simulink model "dig_int_kurt"  (Simulink 6.2)
settings: Solver=ode45  StartTime=0.0  StopTime=1  RelTol=1e-3
undefined symbols (not defined in the file): bit_rev, iBOB, pfb_coeff_gen_calc
libraries: xbsIndex_r3 x1084, casper_library x95, xps_library x32
(part 6 of 8)

== system dig_int_kurt/fft/fft_biplex0/biplex_core/fft_stage_9 ==
  in1 : Inport  Port=1  LatchInput=off
  in2 : Inport  Port=2  LatchInput=off
  of_in : Inport  Port=3  LatchInput=off
  sync : Inport  Port=4  LatchInput=off
  shift : Inport  Port=5  LatchInput=off
  Counter : xbsIndex_r3/Counter  cnt_type=Free Running  n_bits=FFTSize-FFTStage+1  bin_pt=0  arith_type=Unsigned  start_count=0  cnt_to=Inf  cnt_by_val=1  operation=Up  explicit_period=off  period=1  load_pin=off  rst=on  en=off  dbl_ovrd=off  show_param=off  use_rpm=off  gen_core=on
      settings: xl_area=[0, 0, 0, 0, 0, 0, 0]
  Delay : xbsIndex_r3/Delay  latency=1  reg_retiming=off  explicit_period=off  period=1  en=off  accept_only_valid=off  init_zero=on  dbl_ovrd=off  show_param=off
      settings: xl_area=[0, 0, 0, 0, 0, 0, 0]
  Logical1 : xbsIndex_r3/Logical  logical_function=OR  inputs=2  precision=Full  arith_type=Unsigned  n_bits=8  bin_pt=2  align_bp=on  latency=1  explicit_period=on  period=1  en=off  dbl_ovrd=off  show_param=off
      settings: xl_area=[0, 0, 0, 0, 0, 0, 0]
  Mux : xbsIndex_r3/Mux  inputs=2  precision=Full  arith_type="Signed  (2's comp)"  n_bits=8  bin_pt=2  quantization=Truncate  overflow=Wrap  latency=1  explicit_period=off  period=1  en=off  dbl_ovrd=off  show_param=off  mux_type=off  use_rpm=off  gen_core=on
      settings: xl_area=[0, 0, 0, 0, 0, 0, 0]
  Mux1 : xbsIndex_r3/Mux  inputs=2  precision=Full  arith_type="Signed  (2's comp)"  n_bits=8  bin_pt=2  quantization=Truncate  overflow=Wrap  latency=1  explicit_period=off  period=1  en=off  dbl_ovrd=off  show_param=off  mux_type=off  use_rpm=off  gen_core=on
      settings: xl_area=[0, 0, 0, 0, 0, 0, 0]
  Slice : xbsIndex_r3/Slice  Orientation=up  mode=Lower Bit Location + Width  nbits=1  bit1=-(FFTStage - 1)  base1=MSB of Input  bit0=FFTStage - 1  base0=LSB of Input  boolean_output=on  explicit_period=off  period=1  dbl_ovrd=off
  Slice1 : xbsIndex_r3/Slice  mode=Upper Bit Location + Width  nbits=1  bit1=0  base1=MSB of Input  bit0=0  base0=LSB of Input  boolean_output=off  explicit_period=off  period=1  dbl_ovrd=off
  butterfly_direct : Subsystem  AncestorBlock=casper_library/FFTs/butterfly_direct  mask(butterfly_direct){FFTSize=10, Coeffs=getfield( getfield( get_param( gcb,'UserData'), 'parameters'),'Coeffs'), StepPeriod=1, BitWidth=18, add_latency=3, mult_latency=4, bram_latency=3, use_bram=0, quantization=Truncate, overflow=Wrap}
      mask prompts: FFTSize "Size of FFT: (2^?)"; Coeffs "Coefficients: (0 to 2^(FFTSize-1)-1)"; StepPeriod "Coefficient Step Period: (2^?)"; BitWidth "Output Bitwidth:"; add_latency "Add Latency"; mult_latency "Mult Latency"; bram_latency "BRAM Latency"; use_bram "Store Coefficients in BRAM"; quantization "Quantization Behavior"; overflow "Overflow Behavior"
      mask init: same as dig_int_kurt/fft/fft_biplex0/biplex_core/fft_stage_10/butterfly_direct
      settings: AttributesFormatString=|
      | FFTSize=10, Coeffs=[0    1    2    3    4    5    6    7    8    9   10   11   12   13   14   15   16   17   18   19   20   21   22   23   24   25   26   27   28   29   30   31   32   33   34   35   36   37   38   39   40   41   42   43   44   45   46   47   48   49   50   51   52   53   54   55   56   57   58   59   60   61   62   63   64   65   66   67   68   69   70   71   72   73   74   75   76   77   78   79   80   81   82   83   84   85   86   87   88   89   90   91   92   93   94   95   96   97   98   99  100  101  102  103  104  105  106  107  108  109  110  111  112  113  114  115  116  117  118  119  120  121  122  123  124  125  126  127  128  129  130  131  132  133  134  135  136  137  138  139  140  141  142  143  144  145  146  147  148  149  150  151  152  153  154  155  156  157  158  159  160  161  162  163  164  165  166  167  168  169  170  171  172  173  174  175  176  177  178  179  180  181  182  183  184  185  186  187  188  189  190  191  192  193  194  195  196  197  198  199  200  201  202  203  204  205  206  207  208  209  210  211  212  213  214  215  216  217  218  219  220  221  222  223  224  225  226  227  228  229  230  231  232  233  234  235  236  237  238  239  240  241  242  243  244  245  246  247  248  249  250  251  252  253  254  255],
      |  StepPeriod=1, BitWidth=18
      mask StyleString: edit,edit,edit,edit,edit,edit,edit,edit,popup(Truncate|Round  (unbiased: +/- Inf)|Round  (unbiased: Even Values)),popup(Wrap|Saturate|Error)
  delay_b : Subsystem  BlockChoice=delay_slr
      link override delay_bram: bram_latency=bram_latency  DelayLen=2^(FFTSize-FFTStage)
      link override delay_slr: DelayLen=2^(FFTSize-FFTStage)
      settings: AttributesFormatString=%<BlockChoice>  TemplateBlock=casper_library/Delays/delay  MemberBlocks=delay_bram,delay_slr
  delay_f : Subsystem  BlockChoice=delay_slr
      link override delay_bram: bram_latency=bram_latency  DelayLen=2^(FFTSize-FFTStage)
      link override delay_slr: DelayLen=2^(FFTSize-FFTStage)
      settings: AttributesFormatString=%<BlockChoice>  TemplateBlock=casper_library/Delays/delay  MemberBlocks=delay_bram,delay_slr
  sync_delay : casper_library/Delays/sync_delay  DelayLen=2^(FFTSize - FFTStage)
      link override Constant: equ=P=C
      link override Constant1: equ=P=C
      link override Constant2: equ=P=C
      link override Constant3: equ=P=C
  out1 : Outport
  out2 : Outport  Port=2
  of : Outport  Port=3
  sync_out : Outport  Port=4
  wires:
  butterfly_direct/4(sync_out) -> sync_out/1
  butterfly_direct/1(a+bw) -> out1/1
  butterfly_direct/2(a-bw) -> out2/1
  butterfly_direct/3(of) -> Logical1/1
  Slice/1 -> butterfly_direct/4(shift)
  sync_delay/1 -> butterfly_direct/3(sync)
  delay_b/1(Out1) -> butterfly_direct/1(a)
  in2/1 -> delay_f/1(In1)
  Slice1/1 -> Mux1/1, Mux/1
  in1/1 -> Mux1/2, Mux/3
  delay_f/1(Out1) -> Mux/2, Mux1/3
  Mux1/1 -> delay_b/1(In1)
  Mux/1 -> butterfly_direct/2(b)
  Counter/1 -> Slice1/1
  sync/1 -> Delay/1, Counter/1
  Delay/1 -> sync_delay/1
  Logical1/1 -> of/1
  of_in/1 -> Logical1/2
  shift/1 -> Slice/1

== system dig_int_kurt/fft/fft_biplex0/biplex_cplx_unscrambler/barrel_switcher ==
  sel : Inport  Port=1  LatchInput=off
  sync_in : Inport  Port=2  LatchInput=off
  In1 : Inport  Port=3  LatchInput=off
  In2 : Inport  Port=4  LatchInput=off
  Delay_sync : xbsIndex_r3/Delay  latency=1  reg_retiming=off  explicit_period=off  period=1  en=off  accept_only_valid=off  init_zero=on  dbl_ovrd=off  show_param=off
      settings: xl_area=[0, 0, 0, 0, 0, 0, 0]
  Mux11 : xbsIndex_r3/Mux  inputs=2  precision=Full  arith_type="Signed  (2's comp)"  n_bits=8  bin_pt=2  quantization=Truncate  overflow=Wrap  latency=1  explicit_period=off  period=1  en=off  dbl_ovrd=off  show_param=off  mux_type=off  use_rpm=off  gen_core=off
      settings: xl_area=[0, 0, 0, 0, 0, 0, 0]
  Mux21 : xbsIndex_r3/Mux  inputs=2  precision=Full  arith_type="Signed  (2's comp)"  n_bits=8  bin_pt=2  quantization=Truncate  overflow=Wrap  latency=1  explicit_period=off  period=1  en=off  dbl_ovrd=off  show_param=off  mux_type=off  use_rpm=off  gen_core=off
      settings: xl_area=[0, 0, 0, 0, 0, 0, 0]
  Slice1 : xbsIndex_r3/Slice  mode=Upper Bit Location + Width  nbits=1  bit1=-0  base1=MSB of Input  bit0=0  base0=LSB of Input  boolean_output=off  explicit_period=off  period=1  dbl_ovrd=off
  sync_out : Outport
  Out1 : Outport  Port=2
  Out2 : Outport  Port=3
  wires:
  sync_in/1 -> Delay_sync/1
  Delay_sync/1 -> sync_out/1
  sel/1 -> Slice1/1
  Slice1/1 -> Mux11/1, Mux21/1
  In1/1 -> Mux11/2, Mux21/3
  Mux11/1 -> Out1/1
  In2/1 -> Mux21/2, Mux11/3
  Mux21/1 -> Out2/1

== system dig_int_kurt/fft/fft_biplex0/biplex_cplx_unscrambler/barrel_switcher1 ==
  sel : Inport  Port=1  LatchInput=off
  sync_in : Inport  Port=2  LatchInput=off
  In1 : Inport  Port=3  LatchInput=off
  In2 : Inport  Port=4  LatchInput=off
  Delay_sync : xbsIndex_r3/Delay  latency=1  reg_retiming=off  explicit_period=off  period=1  en=off  accept_only_valid=off  init_zero=on  dbl_ovrd=off  show_param=off
      settings: xl_area=[0, 0, 0, 0, 0, 0, 0]
  Mux11 : xbsIndex_r3/Mux  inputs=2  precision=Full  arith_type="Signed  (2's comp)"  n_bits=8  bin_pt=2  quantization=Truncate  overflow=Wrap  latency=1  explicit_period=off  period=1  en=off  dbl_ovrd=off  show_param=off  mux_type=off  use_rpm=off  gen_core=off
      settings: xl_area=[0, 0, 0, 0, 0, 0, 0]
  Mux21 : xbsIndex_r3/Mux  inputs=2  precision=Full  arith_type="Signed  (2's comp)"  n_bits=8  bin_pt=2  quantization=Truncate  overflow=Wrap  latency=1  explicit_period=off  period=1  en=off  dbl_ovrd=off  show_param=off  mux_type=off  use_rpm=off  gen_core=off
      settings: xl_area=[0, 0, 0, 0, 0, 0, 0]
  Slice1 : xbsIndex_r3/Slice  mode=Upper Bit Location + Width  nbits=1  bit1=-0  base1=MSB of Input  bit0=0  base0=LSB of Input  boolean_output=off  explicit_period=off  period=1  dbl_ovrd=off
  sync_out : Outport
  Out1 : Outport  Port=2
  Out2 : Outport  Port=3
  wires:
  sync_in/1 -> Delay_sync/1
  Delay_sync/1 -> sync_out/1
  sel/1 -> Slice1/1
  Slice1/1 -> Mux11/1, Mux21/1
  In1/1 -> Mux11/2, Mux21/3
  Mux11/1 -> Out1/1
  In2/1 -> Mux21/2, Mux11/3
  Mux21/1 -> Out2/1

== system dig_int_kurt/fft/fft_biplex0/biplex_cplx_unscrambler/reorder ==
  sync : Inport  Port=1  LatchInput=off
  en : Inport  Port=2  LatchInput=off
  din0 : Inport  Port=3  LatchInput=off
  Counter : xbsIndex_r3/Counter  cnt_type=Count Limited  n_bits=11  bin_pt=0  arith_type=Unsigned  start_count=0  cnt_to=2047  cnt_by_val=1  operation=Up  explicit_period=off  period=1  load_pin=off  rst=on  en=on  dbl_ovrd=off  show_param=off  use_rpm=on  gen_core=off
      settings: xl_area=[0, 0, 0, 0, 0, 0, 0]
  Mux : xbsIndex_r3/Mux  inputs=2  precision=Full  arith_type="Signed  (2's comp)"  n_bits=8  bin_pt=2  quantization=Truncate  overflow=Wrap  latency=1  explicit_period=off  period=1  en=off  dbl_ovrd=off  show_param=off  mux_type=off  use_rpm=off  gen_core=off
      settings: xl_area=[0, 0, 0, 0, 0, 0, 0]
  Slice1 : xbsIndex_r3/Slice  mode=Upper Bit Location + Width  nbits=1  bit1=0  base1=MSB of Input  bit0=0  base0=LSB of Input  boolean_output=off  explicit_period=off  period=1  dbl_ovrd=off
  Slice2 : xbsIndex_r3/Slice  mode=Lower Bit Location + Width  nbits=10  bit1=0  base1=MSB of Input  bit0=0  base0=LSB of Input  boolean_output=off  explicit_period=off  period=1  dbl_ovrd=off
  bram0 : xbsIndex_r3/Single Port RAM  depth=1024  initVector=sin(pi*(0:15)/16)  write_mode=Read Before Write  latency=3  init_zero=on  explicit_period=off  period=1  rst=off  init_reg=0  en=off  dbl_ovrd=off  show_param=off  distributed_mem=off  use_rpm=off  gen_core=off
      settings: xl_area=[0, 0, 0, 0, 0, 0, 0]
  delay_d0 : xbsIndex_r3/Delay  latency=0  reg_retiming=off  explicit_period=off  period=1  en=off  accept_only_valid=off  init_zero=on  dbl_ovrd=off  show_param=off
      settings: xl_area=[0, 0, 0, 0, 0, 0, 0]
  delay_din0 : xbsIndex_r3/Delay  latency=1  reg_retiming=off  explicit_period=off  period=1  en=off  accept_only_valid=off  init_zero=on  dbl_ovrd=off  show_param=off
      settings: xl_area=[0, 0, 0, 0, 0, 0, 0]
  delay_map1 : xbsIndex_r3/Delay  latency=0*map_latency  reg_retiming=off  explicit_period=off  period=1  en=off  accept_only_valid=off  init_zero=on  dbl_ovrd=off  show_param=off
      settings: xl_area=[0, 0, 0, 0, 0, 0, 0]
  delay_sel : xbsIndex_r3/Delay  latency=0  reg_retiming=off  explicit_period=off  period=1  en=off  accept_only_valid=off  init_zero=on  dbl_ovrd=off  show_param=off
      settings: xl_area=[0, 0, 0, 0, 0, 0, 0]
  delay_valid : xbsIndex_r3/Delay  latency=4  reg_retiming=off  explicit_period=off  period=1  en=off  accept_only_valid=off  init_zero=on  dbl_ovrd=off  show_param=off
      settings: xl_area=[0, 0, 0, 0, 0, 0, 0]
  delay_we : xbsIndex_r3/Delay  latency=0  reg_retiming=off  explicit_period=off  period=1  en=off  accept_only_valid=off  init_zero=on  dbl_ovrd=off  show_param=off
      settings: xl_area=[0, 0, 0, 0, 0, 0, 0]
  map1 : Subsystem  AncestorBlock=casper_library/FFTs/map  mask(map){map=getfield( getfield( get_param( gcb,'UserData'), 'parameters'),'map'), latency=0}
      mask init:
      | map_init(gcb, 'map', map, 'latency', latency)
  post_sync_delay : xbsIndex_r3/Delay  latency=4  reg_retiming=off  explicit_period=off  period=1  en=off  accept_only_valid=off  init_zero=on  dbl_ovrd=off  show_param=off
      settings: xl_area=[0, 0, 0, 0, 0, 0, 0]
  pre_sync_delay : xbsIndex_r3/Delay  latency=0  reg_retiming=off  explicit_period=off  period=1  en=off  accept_only_valid=off  init_zero=on  dbl_ovrd=off  show_param=off
      settings: xl_area=[0, 0, 0, 0, 0, 0, 0]
  sync_delay_en : casper_library/Delays/sync_delay_en  DelayLen=1024
      link override Constant: equ=P=C
      link override Constant1: equ=P=C
      link override Constant2: equ=P=C
      link override Constant3: equ=P=C
  sync_out : Outport
  valid : Outport  Port=2
  dout0 : Outport  Port=3
  wires:
  sync/1 -> Counter/1, pre_sync_delay/1
  en/1 -> Counter/2, sync_delay_en/2, delay_we/1
  Counter/1 -> Slice1/1, Slice2/1
  Slice1/1 -> delay_sel/1
  delay_sel/1 -> Mux/1
  Slice2/1 -> delay_d0/1, map1/1(din)
  delay_d0/1 -> Mux/2
  pre_sync_delay/1 -> sync_delay_en/1
  sync_delay_en/1 -> post_sync_delay/1
  post_sync_delay/1 -> sync_out/1
  delay_we/1 -> delay_valid/1, bram0/3
  delay_valid/1 -> valid/1
  Mux/1 -> bram0/1
  din0/1 -> delay_din0/1
  delay_din0/1 -> bram0/2
  bram0/1 -> dout0/1
  map1/1(dout) -> delay_map1/1
  delay_map1/1 -> Mux/3

== system dig_int_kurt/fft/fft_biplex0/biplex_cplx_unscrambler/reorder1 ==
  sync : Inport  Port=1  LatchInput=off
  en : Inport  Port=2  LatchInput=off
  din0 : Inport  Port=3  LatchInput=off
  Counter : xbsIndex_r3/Counter  cnt_type=Count Limited  n_bits=11  bin_pt=0  arith_type=Unsigned  start_count=0  cnt_to=2047  cnt_by_val=1  operation=Up  explicit_period=off  period=1  load_pin=off  rst=on  en=on  dbl_ovrd=off  show_param=off  use_rpm=on  gen_core=off
      settings: xl_area=[0, 0, 0, 0, 0, 0, 0]
  Mux : xbsIndex_r3/Mux  inputs=2  precision=Full  arith_type="Signed  (2's comp)"  n_bits=8  bin_pt=2  quantization=Truncate  overflow=Wrap  latency=1  explicit_period=off  period=1  en=off  dbl_ovrd=off  show_param=off  mux_type=off  use_rpm=off  gen_core=off
      settings: xl_area=[0, 0, 0, 0, 0, 0, 0]
  Slice1 : xbsIndex_r3/Slice  mode=Upper Bit Location + Width  nbits=1  bit1=0  base1=MSB of Input  bit0=0  base0=LSB of Input  boolean_output=off  explicit_period=off  period=1  dbl_ovrd=off
  Slice2 : xbsIndex_r3/Slice  mode=Lower Bit Location + Width  nbits=10  bit1=0  base1=MSB of Input  bit0=0  base0=LSB of Input  boolean_output=off  explicit_period=off  period=1  dbl_ovrd=off
  bram0 : xbsIndex_r3/Single Port RAM  depth=1024  initVector=sin(pi*(0:15)/16)  write_mode=Read Before Write  latency=3  init_zero=on  explicit_period=off  period=1  rst=off  init_reg=0  en=off  dbl_ovrd=off  show_param=off  distributed_mem=off  use_rpm=off  gen_core=off
      settings: xl_area=[0, 0, 0, 0, 0, 0, 0]
  delay_d0 : xbsIndex_r3/Delay  latency=0  reg_retiming=off  explicit_period=off  period=1  en=off  accept_only_valid=off  init_zero=on  dbl_ovrd=off  show_param=off
      settings: xl_area=[0, 0, 0, 0, 0, 0, 0]
  delay_din0 : xbsIndex_r3/Delay  latency=1  reg_retiming=off  explicit_period=off  period=1  en=off  accept_only_valid=off  init_zero=on  dbl_ovrd=off  show_param=off
      settings: xl_area=[0, 0, 0, 0, 0, 0, 0]
  delay_map1 : xbsIndex_r3/Delay  latency=0*map_latency  reg_retiming=off  explicit_period=off  period=1  en=off  accept_only_valid=off  init_zero=on  dbl_ovrd=off  show_param=off
      settings: xl_area=[0, 0, 0, 0, 0, 0, 0]
  delay_sel : xbsIndex_r3/Delay  latency=0  reg_retiming=off  explicit_period=off  period=1  en=off  accept_only_valid=off  init_zero=on  dbl_ovrd=off  show_param=off
      settings: xl_area=[0, 0, 0, 0, 0, 0, 0]
  delay_valid : xbsIndex_r3/Delay  latency=4  reg_retiming=off  explicit_period=off  period=1  en=off  accept_only_valid=off  init_zero=on  dbl_ovrd=off  show_param=off
      settings: xl_area=[0, 0, 0, 0, 0, 0, 0]
  delay_we : xbsIndex_r3/Delay  latency=0  reg_retiming=off  explicit_period=off  period=1  en=off  accept_only_valid=off  init_zero=on  dbl_ovrd=off  show_param=off
      settings: xl_area=[0, 0, 0, 0, 0, 0, 0]
  map1 : Subsystem  AncestorBlock=casper_library/FFTs/map  mask(map){map=getfield( getfield( get_param( gcb,'UserData'), 'parameters'),'map'), latency=0}
      mask init:
      | map_init(gcb, 'map', map, 'latency', latency)
  post_sync_delay : xbsIndex_r3/Delay  latency=4  reg_retiming=off  explicit_period=off  period=1  en=off  accept_only_valid=off  init_zero=on  dbl_ovrd=off  show_param=off
      settings: xl_area=[0, 0, 0, 0, 0, 0, 0]
  pre_sync_delay : xbsIndex_r3/Delay  latency=0  reg_retiming=off  explicit_period=off  period=1  en=off  accept_only_valid=off  init_zero=on  dbl_ovrd=off  show_param=off
      settings: xl_area=[0, 0, 0, 0, 0, 0, 0]
  sync_delay_en : casper_library/Delays/sync_delay_en  DelayLen=1024
      link override Constant: equ=P=C
      link override Constant1: equ=P=C
      link override Constant2: equ=P=C
      link override Constant3: equ=P=C
  sync_out : Outport
  valid : Outport  Port=2
  dout0 : Outport  Port=3
  wires:
  sync/1 -> Counter/1, pre_sync_delay/1
  en/1 -> Counter/2, sync_delay_en/2, delay_we/1
  Counter/1 -> Slice1/1, Slice2/1
  Slice1/1 -> delay_sel/1
  delay_sel/1 -> Mux/1
  Slice2/1 -> delay_d0/1, map1/1(din)
  delay_d0/1 -> Mux/2
  pre_sync_delay/1 -> sync_delay_en/1
  sync_delay_en/1 -> post_sync_delay/1
  post_sync_delay/1 -> sync_out/1
  delay_we/1 -> delay_valid/1, bram0/3
  delay_valid/1 -> valid/1
  Mux/1 -> bram0/1
  din0/1 -> delay_din0/1
  delay_din0/1 -> bram0/2
  bram0/1 -> dout0/1
  map1/1(dout) -> delay_map1/1
  delay_map1/1 -> Mux/3

== system dig_int_kurt/pfb_fir/pol1_in1_last_tap/pfb_add_tree/adder_tree1 ==
  sync : Inport  Port=1  LatchInput=off
  din1 : Inport  Port=2  LatchInput=off
  din2 : Inport  Port=3  LatchInput=off
  din3 : Inport  Port=4  LatchInput=off
  din4 : Inport  Port=5  LatchInput=off
  addr1 : xbsIndex_r3/AddSub  mode=Addition  precision=Full  arith_type=Unsigned  n_bits=8  bin_pt=2  quantization=Truncate  overflow=Wrap  latency=2  explicit_period=off  period=1  use_carryin=off  use_carryout=off  en=off  dbl_ovrd=off  show_param=off  use_core=on  pipeline=on  use_rpm=on  gen_core=off
      settings: xl_area=[0, 0, 0, 0, 0, 0, 0]
  addr2 : xbsIndex_r3/AddSub  mode=Addition  precision=Full  arith_type=Unsigned  n_bits=8  bin_pt=2  quantization=Truncate  overflow=Wrap  latency=2  explicit_period=off  period=1  use_carryin=off  use_carryout=off  en=off  dbl_ovrd=off  show_param=off  use_core=on  pipeline=on  use_rpm=on  gen_core=off
      settings: xl_area=[0, 0, 0, 0, 0, 0, 0]
  addr3 : xbsIndex_r3/AddSub  mode=Addition  precision=Full  arith_type=Unsigned  n_bits=8  bin_pt=2  quantization=Truncate  overflow=Wrap  latency=2  explicit_period=off  period=1  use_carryin=off  use_carryout=off  en=off  dbl_ovrd=off  show_param=off  use_core=on  pipeline=on  use_rpm=on  gen_core=off
      settings: xl_area=[0, 0, 0, 0, 0, 0, 0]
  sync_delay : xbsIndex_r3/Delay  latency=4  reg_retiming=off  explicit_period=off  period=1  en=off  accept_only_valid=off  init_zero=on  dbl_ovrd=off  show_param=off
      settings: xl_area=[0, 0, 0, 0, 0, 0, 0]
  sync_out : Outport
  dout : Outport  Port=2
  wires:
  sync/1 -> sync_delay/1
  sync_delay/1 -> sync_out/1
  din1/1 -> addr1/1
  din2/1 -> addr1/2
  din3/1 -> addr2/1
  din4/1 -> addr2/2
  addr1/1 -> addr3/1
  addr2/1 -> addr3/2
  addr3/1 -> dout/1

== system dig_int_kurt/pfb_fir/pol1_in1_last_tap/pfb_add_tree/adder_tree2 ==
  sync : Inport  Port=1  LatchInput=off
  din1 : Inport  Port=2  LatchInput=off
  din2 : Inport  Port=3  LatchInput=off
  din3 : Inport  Port=4  LatchInput=off
  din4 : Inport  Port=5  LatchInput=off
  addr1 : xbsIndex_r3/AddSub  mode=Addition  precision=Full  arith_type=Unsigned  n_bits=8  bin_pt=2  quantization=Truncate  overflow=Wrap  latency=2  explicit_period=off  period=1  use_carryin=off  use_carryout=off  en=off  dbl_ovrd=off  show_param=off  use_core=on  pipeline=on  use_rpm=on  gen_core=off
      settings: xl_area=[0, 0, 0, 0, 0, 0, 0]
  addr2 : xbsIndex_r3/AddSub  mode=Addition  precision=Full  arith_type=Unsigned  n_bits=8  bin_pt=2  quantization=Truncate  overflow=Wrap  latency=2  explicit_period=off  period=1  use_carryin=off  use_carryout=off  en=off  dbl_ovrd=off  show_param=off  use_core=on  pipeline=on  use_rpm=on  gen_core=off
      settings: xl_area=[0, 0, 0, 0, 0, 0, 0]
  addr3 : xbsIndex_r3/AddSub  mode=Addition  precision=Full  arith_type=Unsigned  n_bits=8  bin_pt=2  quantization=Truncate  overflow=Wrap  latency=2  explicit_period=off  period=1  use_carryin=off  use_carryout=off  en=off  dbl_ovrd=off  show_param=off  use_core=on  pipeline=on  use_rpm=on  gen_core=off
      settings: xl_area=[0, 0, 0, 0, 0, 0, 0]
  sync_delay : xbsIndex_r3/Delay  latency=4  reg_retiming=off  explicit_period=off  period=1  en=off  accept_only_valid=off  init_zero=on  dbl_ovrd=off  show_param=off
      settings: xl_area=[0, 0, 0, 0, 0, 0, 0]
  sync_out : Outport
  dout : Outport  Port=2
  wires:
  sync/1 -> sync_delay/1
  sync_delay/1 -> sync_out/1
  din1/1 -> addr1/1
  din2/1 -> addr1/2
  din3/1 -> addr2/1
  din4/1 -> addr2/2
  addr1/1 -> addr3/1
  addr2/1 -> addr3/2
  addr3/1 -> dout/1

== system dig_int_kurt/pfb_fir/pol2_in1_last_tap/pfb_add_tree/adder_tree1 ==
  sync : Inport  Port=1  LatchInput=off
  din1 : Inport  Port=2  LatchInput=off
  din2 : Inport  Port=3  LatchInput=off
  din3 : Inport  Port=4  LatchInput=off
  din4 : Inport  Port=5  LatchInput=off
  addr1 : xbsIndex_r3/AddSub  mode=Addition  precision=Full  arith_type=Unsigned  n_bits=8  bin_pt=2  quantization=Truncate  overflow=Wrap  latency=2  explicit_period=off  period=1  use_carryin=off  use_carryout=off  en=off  dbl_ovrd=off  show_param=off  use_core=on  pipeline=on  use_rpm=on  gen_core=off
      settings: xl_area=[0, 0, 0, 0, 0, 0, 0]
  addr2 : xbsIndex_r3/AddSub  mode=Addition  precision=Full  arith_type=Unsigned  n_bits=8  bin_pt=2  quantization=Truncate  overflow=Wrap  latency=2  explicit_period=off  period=1  use_carryin=off  use_carryout=off  en=off  dbl_ovrd=off  show_param=off  use_core=on  pipeline=on  use_rpm=on  gen_core=off
      settings: xl_area=[0, 0, 0, 0, 0, 0, 0]
  addr3 : xbsIndex_r3/AddSub  mode=Addition  precision=Full  arith_type=Unsigned  n_bits=8  bin_pt=2  quantization=Truncate  overflow=Wrap  latency=2  explicit_period=off  period=1  use_carryin=off  use_carryout=off  en=off  dbl_ovrd=off  show_param=off  use_core=on  pipeline=on  use_rpm=on  gen_core=off
      settings: xl_area=[0, 0, 0, 0, 0, 0, 0]
  sync_delay : xbsIndex_r3/Delay  latency=4  reg_retiming=off  explicit_period=off  period=1  en=off  accept_only_valid=off  init_zero=on  dbl_ovrd=off  show_param=off
      settings: xl_area=[0, 0, 0, 0, 0, 0, 0]
  sync_out : Outport
  dout : Outport  Port=2
  wires:
  sync/1 -> sync_delay/1
  sync_delay/1 -> sync_out/1
  din1/1 -> addr1/1
  din2/1 -> addr1/2
  din3/1 -> addr2/1
  din4/1 -> addr2/2
  addr1/1 -> addr3/1
  addr2/1 -> addr3/2
  addr3/1 -> dout/1

== system dig_int_kurt/pfb_fir/pol2_in1_last_tap/pfb_add_tree/adder_tree2 ==
  sync : Inport  Port=1  LatchInput=off
  din1 : Inport  Port=2  LatchInput=off
  din2 : Inport  Port=3  LatchInput=off
  din3 : Inport  Port=4  LatchInput=off
  din4 : Inport  Port=5  LatchInput=off
  addr1 : xbsIndex_r3/AddSub  mode=Addition  precision=Full  arith_type=Unsigned  n_bits=8  bin_pt=2  quantization=Truncate  overflow=Wrap  latency=2  explicit_period=off  period=1  use_carryin=off  use_carryout=off  en=off  dbl_ovrd=off  show_param=off  use_core=on  pipeline=on  use_rpm=on  gen_core=off
      settings: xl_area=[0, 0, 0, 0, 0, 0, 0]
  addr2 : xbsIndex_r3/AddSub  mode=Addition  precision=Full  arith_type=Unsigned  n_bits=8  bin_pt=2  quantization=Truncate  overflow=Wrap  latency=2  explicit_period=off  period=1  use_carryin=off  use_carryout=off  en=off  dbl_ovrd=off  show_param=off  use_core=on  pipeline=on  use_rpm=on  gen_core=off
      settings: xl_area=[0, 0, 0, 0, 0, 0, 0]
  addr3 : xbsIndex_r3/AddSub  mode=Addition  precision=Full  arith_type=Unsigned  n_bits=8  bin_pt=2  quantization=Truncate  overflow=Wrap  latency=2  explicit_period=off  period=1  use_carryin=off  use_carryout=off  en=off  dbl_ovrd=off  show_param=off  use_core=on  pipeline=on  use_rpm=on  gen_core=off
      settings: xl_area=[0, 0, 0, 0, 0, 0, 0]
  sync_delay : xbsIndex_r3/Delay  latency=4  reg_retiming=off  explicit_period=off  period=1  en=off  accept_only_valid=off  init_zero=on  dbl_ovrd=off  show_param=off
      settings: xl_area=[0, 0, 0, 0, 0, 0, 0]
  sync_out : Outport
  dout : Outport  Port=2
  wires:
  sync/1 -> sync_delay/1
  sync_delay/1 -> sync_out/1
  din1/1 -> addr1/1
  din2/1 -> addr1/2
  din3/1 -> addr2/1
  din4/1 -> addr2/2
  addr1/1 -> addr3/1
  addr2/1 -> addr3/2
  addr3/1 -> dout/1

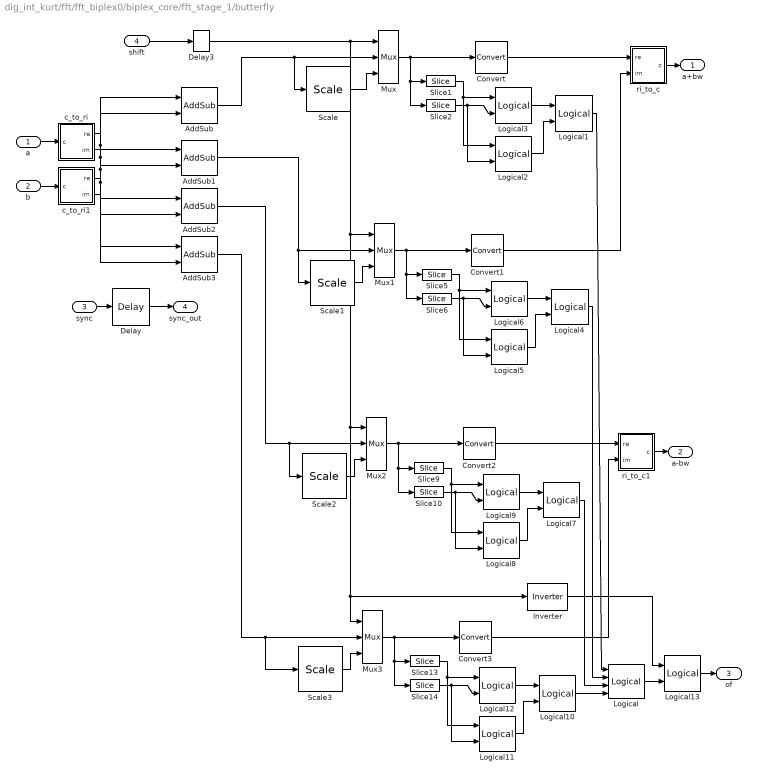
== system dig_int_kurt/fft/fft_biplex0/biplex_core/fft_stage_1/butterfly ==
  a : Inport  Port=1  LatchInput=off
  b : Inport  Port=2  LatchInput=off
  sync : Inport  Port=3  LatchInput=off
  shift : Inport  Port=4  LatchInput=off
  AddSub : xbsIndex_r3/AddSub  mode=Addition  precision=Full  arith_type=Unsigned  n_bits=8  bin_pt=2  quantization=Truncate  overflow=Wrap  latency=add_latency  explicit_period=off  period=1  use_carryin=off  use_carryout=off  en=off  dbl_ovrd=off  show_param=on  use_core=on  pipeline=on  use_rpm=on  gen_core=on
      settings: xl_area=[0, 0, 0, 0, 0, 0, 0]
  AddSub1 : xbsIndex_r3/AddSub  mode=Addition  precision=Full  arith_type=Unsigned  n_bits=8  bin_pt=2  quantization=Truncate  overflow=Wrap  latency=add_latency  explicit_period=off  period=1  use_carryin=off  use_carryout=off  en=off  dbl_ovrd=off  show_param=on  use_core=on  pipeline=on  use_rpm=on  gen_core=on
      settings: xl_area=[0, 0, 0, 0, 0, 0, 0]
  AddSub2 : xbsIndex_r3/AddSub  mode=Subtraction  precision=Full  arith_type=Unsigned  n_bits=8  bin_pt=2  quantization=Truncate  overflow=Wrap  latency=add_latency  explicit_period=off  period=1  use_carryin=off  use_carryout=off  en=off  dbl_ovrd=off  show_param=on  use_core=on  pipeline=on  use_rpm=on  gen_core=on
      settings: xl_area=[0, 0, 0, 0, 0, 0, 0]
  AddSub3 : xbsIndex_r3/AddSub  mode=Subtraction  precision=Full  arith_type=Unsigned  n_bits=8  bin_pt=2  quantization=Truncate  overflow=Wrap  latency=add_latency  explicit_period=off  period=1  use_carryin=off  use_carryout=off  en=off  dbl_ovrd=off  show_param=on  use_core=on  pipeline=on  use_rpm=on  gen_core=on
      settings: xl_area=[0, 0, 0, 0, 0, 0, 0]
  Convert{,1..3} (4 alike) : xbsIndex_r3/Convert  arith_type="Signed  (2's comp)"  n_bits=BitWidth  bin_pt=BitWidth-1  quantization=Truncate  overflow=Wrap  latency=add_latency  explicit_period=off  period=1  dbl_ovrd=off  show_param=off  inserted_by_tool=off  pipeline=off
      settings: xl_area=[0, 0, 0, 0, 0, 0, 0]
  Delay : xbsIndex_r3/Delay  latency=2 * add_latency + 1  reg_retiming=off  explicit_period=off  period=1  en=off  accept_only_valid=off  init_zero=on  dbl_ovrd=off  show_param=off
      settings: xl_area=[0, 0, 0, 0, 0, 0, 0]
  Delay3 : xbsIndex_r3/Delay  latency=1  reg_retiming=off  explicit_period=off  period=1  en=off  accept_only_valid=off  init_zero=on  dbl_ovrd=off  show_param=off
      settings: xl_area=[0, 0, 0, 0, 0, 0, 0]
  Inverter : xbsIndex_r3/Inverter  latency=0  explicit_period=off  period=1  en=off  dbl_ovrd=off  show_param=off
      settings: xl_area=[0, 0, 0, 0, 0, 0, 0]
  Logical : xbsIndex_r3/Logical  logical_function=OR  inputs=4  precision=Full  arith_type=Unsigned  n_bits=8  bin_pt=2  align_bp=on  latency=1  explicit_period=off  period=1  en=off  dbl_ovrd=off  show_param=off
      settings: xl_area=[0, 0, 0, 0, 0, 0, 0]
  Logical{1,4,7,10} (4 alike) : xbsIndex_r3/Logical  logical_function=OR  inputs=2  precision=Full  arith_type=Unsigned  n_bits=8  bin_pt=2  align_bp=off  latency=1  explicit_period=off  period=1  en=off  dbl_ovrd=off  show_param=off
      settings: xl_area=[0, 0, 0, 0, 0, 0, 0]
  Logical{2,5,8,11} (4 alike) : xbsIndex_r3/Logical  logical_function=NOR  inputs=2  precision=Full  arith_type=Unsigned  n_bits=8  bin_pt=2  align_bp=off  latency=1  explicit_period=off  period=1  en=off  dbl_ovrd=off  show_param=off
      settings: xl_area=[0, 0, 0, 0, 0, 0, 0]
  Logical{3,6,9,12..13} (5 alike) : xbsIndex_r3/Logical  logical_function=AND  inputs=2  precision=Full  arith_type=Unsigned  n_bits=8  bin_pt=2  align_bp=off  latency=1  explicit_period=off  period=1  en=off  dbl_ovrd=off  show_param=off
      settings: xl_area=[0, 0, 0, 0, 0, 0, 0]
  Mux{,1..3} (4 alike) : xbsIndex_r3/Mux  inputs=2  precision=Full  arith_type="Signed  (2's comp)"  n_bits=8  bin_pt=2  quantization=Truncate  overflow=Wrap  latency=1  explicit_period=off  period=1  en=off  dbl_ovrd=off  show_param=off  mux_type=off  use_rpm=off  gen_core=off
      settings: xl_area=[0, 0, 0, 0, 0, 0, 0]
  Scale{,1..3} (4 alike) : xbsIndex_r3/Scale  scale_factor=-1  explicit_period=off  period=1  dbl_ovrd=off
  Slice{1,5,9,13} (4 alike) : xbsIndex_r3/Slice  mode=Upper Bit Location + Width  nbits=1  bit1=0  base1=MSB of Input  bit0=0  base0=LSB of Input  boolean_output=on  explicit_period=off  period=1  dbl_ovrd=off
  Slice{2,6,10,14} (4 alike) : xbsIndex_r3/Slice  mode=Upper Bit Location + Width  nbits=1  bit1=-1  base1=MSB of Input  bit0=0  base0=LSB of Input  boolean_output=on  explicit_period=off  period=1  dbl_ovrd=off
  c_to_ri : Subsystem
  c_to_ri1 : Subsystem
  ri_to_c : Subsystem
  ri_to_c1 : Subsystem
  a+bw : Outport
  a-bw : Outport  Port=2
  of : Outport  Port=3
  sync_out : Outport  Port=4
  wires:
  b/1 -> c_to_ri1/1(c)
  a/1 -> c_to_ri/1(c)
  sync/1 -> Delay/1
  c_to_ri1/2(im) -> AddSub3/2, AddSub1/2
  c_to_ri1/1(re) -> AddSub2/2, AddSub/2
  c_to_ri/2(im) -> AddSub3/1, AddSub1/1
  c_to_ri/1(re) -> AddSub2/1, AddSub/1
  ri_to_c/1(c) -> a+bw/1
  ri_to_c1/1(c) -> a-bw/1
  Delay/1 -> sync_out/1
  AddSub/1 -> Mux/2, Scale/1
  AddSub1/1 -> Mux1/2, Scale1/1
  shift/1 -> Delay3/1
  Mux/1 -> Convert/1, Slice2/1, Slice1/1
  Scale/1 -> Mux/3
  Convert/1 -> ri_to_c/1(re)
  Slice1/1 -> Logical3/1, Logical2/1
  Slice2/1 -> Logical3/2, Logical2/2
  Logical3/1 -> Logical1/1
  Logical2/1 -> Logical1/2
  Logical1/1 -> Logical/1
  Mux1/1 -> Convert1/1, Slice6/1, Slice5/1
  Scale1/1 -> Mux1/3
  Convert1/1 -> ri_to_c/2(im)
  Slice5/1 -> Logical6/1, Logical5/1
  Slice6/1 -> Logical6/2, Logical5/2
  Logical6/1 -> Logical4/1
  Logical5/1 -> Logical4/2
  Logical4/1 -> Logical/2
  Mux2/1 -> Convert2/1, Slice10/1, Slice9/1
  Scale2/1 -> Mux2/3
  Convert2/1 -> ri_to_c1/1(re)
  Slice9/1 -> Logical9/1, Logical8/1
  Slice10/1 -> Logical9/2, Logical8/2
  Logical9/1 -> Logical7/1
  Logical8/1 -> Logical7/2
  AddSub2/1 -> Mux2/2, Scale2/1
  Mux3/1 -> Convert3/1, Slice14/1, Slice13/1
  Scale3/1 -> Mux3/3
  Convert3/1 -> ri_to_c1/2(im)
  Slice13/1 -> Logical12/1, Logical11/1
  Slice14/1 -> Logical12/2, Logical11/2
  Logical12/1 -> Logical10/1
  Logical11/1 -> Logical10/2
  Logical10/1 -> Logical/4
  AddSub3/1 -> Mux3/2, Scale3/1
  Logical7/1 -> Logical/3
  Delay3/1 -> Mux/1, Mux1/1, Mux2/1, Mux3/1, Inverter/1
  Logical/1 -> Logical13/2
  Logical13/1 -> of/1
  Inverter/1 -> Logical13/1

== system dig_int_kurt/fft/fft_biplex0/biplex_core/fft_stage_1/delay_b ==
  In1 : Inport  Port=1  LatchInput=off
  delay_bram : casper_library/Delays/delay_bram  DelayLen=2^(FFTSize-FFTStage)  bram_latency=bram_latency
  Out1 : Outport
  wires:
  In1/1 -> delay_bram/1
  delay_bram/1 -> Out1/1

== system dig_int_kurt/fft/fft_biplex0/biplex_core/fft_stage_1/delay_f ==
  In1 : Inport  Port=1  LatchInput=off
  delay_bram : casper_library/Delays/delay_bram  DelayLen=2^(FFTSize-FFTStage)  bram_latency=bram_latency
  Out1 : Outport
  wires:
  In1/1 -> delay_bram/1
  delay_bram/1 -> Out1/1

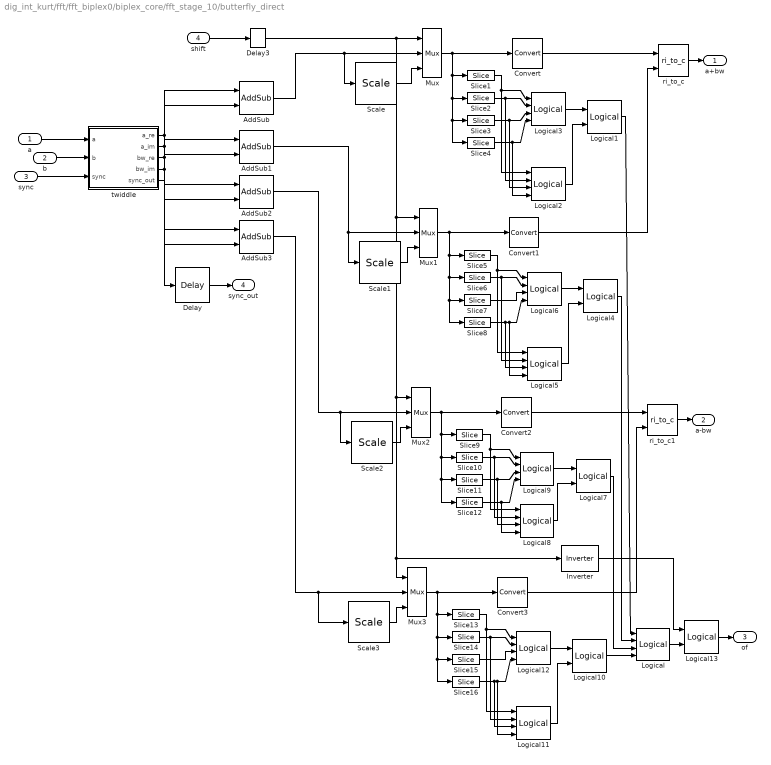
== system dig_int_kurt/fft/fft_biplex0/biplex_core/fft_stage_10/butterfly_direct ==
  a : Inport  Port=1  LatchInput=off
  b : Inport  Port=2  LatchInput=off
  sync : Inport  Port=3  LatchInput=off
  shift : Inport  Port=4  LatchInput=off
  AddSub : xbsIndex_r3/AddSub  mode=Addition  precision=Full  arith_type=Unsigned  n_bits=8  bin_pt=2  quantization=Truncate  overflow=Wrap  latency=add_latency  explicit_period=off  period=1  use_carryin=off  use_carryout=off  en=off  dbl_ovrd=off  show_param=on  use_core=on  pipeline=on  use_rpm=on  gen_core=on
      settings: xl_area=[0, 0, 0, 0, 0, 0, 0]
  AddSub1 : xbsIndex_r3/AddSub  mode=Addition  precision=Full  arith_type=Unsigned  n_bits=8  bin_pt=2  quantization=Truncate  overflow=Wrap  latency=add_latency  explicit_period=off  period=1  use_carryin=off  use_carryout=off  en=off  dbl_ovrd=off  show_param=on  use_core=on  pipeline=on  use_rpm=on  gen_core=on
      settings: xl_area=[0, 0, 0, 0, 0, 0, 0]
  AddSub2 : xbsIndex_r3/AddSub  mode=Subtraction  precision=Full  arith_type=Unsigned  n_bits=8  bin_pt=2  quantization=Truncate  overflow=Wrap  latency=add_latency  explicit_period=off  period=1  use_carryin=off  use_carryout=off  en=off  dbl_ovrd=off  show_param=on  use_core=on  pipeline=on  use_rpm=on  gen_core=on
      settings: xl_area=[0, 0, 0, 0, 0, 0, 0]
  AddSub3 : xbsIndex_r3/AddSub  mode=Subtraction  precision=Full  arith_type=Unsigned  n_bits=8  bin_pt=2  quantization=Truncate  overflow=Wrap  latency=add_latency  explicit_period=off  period=1  use_carryin=off  use_carryout=off  en=off  dbl_ovrd=off  show_param=on  use_core=on  pipeline=on  use_rpm=on  gen_core=on
      settings: xl_area=[0, 0, 0, 0, 0, 0, 0]
  Convert{,1..3} (4 alike) : xbsIndex_r3/Convert  arith_type="Signed  (2's comp)"  n_bits=BitWidth  bin_pt=BitWidth-1  quantization=Truncate  overflow=Wrap  latency=add_latency  explicit_period=off  period=1  dbl_ovrd=off  show_param=off  inserted_by_tool=off  pipeline=off
      settings: xl_area=[0, 0, 0, 0, 0, 0, 0]
  Delay : xbsIndex_r3/Delay  latency=2 * add_latency + 1  reg_retiming=off  explicit_period=off  period=1  en=off  accept_only_valid=off  init_zero=on  dbl_ovrd=off  show_param=off
      settings: xl_area=[0, 0, 0, 0, 0, 0, 0]
  Delay3 : xbsIndex_r3/Delay  latency=1  reg_retiming=off  explicit_period=off  period=1  en=off  accept_only_valid=off  init_zero=on  dbl_ovrd=off  show_param=off
      settings: xl_area=[0, 0, 0, 0, 0, 0, 0]
  Inverter : xbsIndex_r3/Inverter  latency=0  explicit_period=off  period=1  en=off  dbl_ovrd=off  show_param=off
      settings: xl_area=[0, 0, 0, 0, 0, 0, 0]
  Logical : xbsIndex_r3/Logical  logical_function=OR  inputs=4  precision=Full  arith_type=Unsigned  n_bits=8  bin_pt=2  align_bp=on  latency=1  explicit_period=off  period=1  en=off  dbl_ovrd=off  show_param=off
      settings: xl_area=[0, 0, 0, 0, 0, 0, 0]
  Logical{1,4,7,10} (4 alike) : xbsIndex_r3/Logical  logical_function=OR  inputs=2  precision=Full  arith_type=Unsigned  n_bits=8  bin_pt=2  align_bp=off  latency=1  explicit_period=off  period=1  en=off  dbl_ovrd=off  show_param=off
      settings: xl_area=[0, 0, 0, 0, 0, 0, 0]
  Logical{2,5,8,11} (4 alike) : xbsIndex_r3/Logical  logical_function=NOR  inputs=4  precision=Full  arith_type=Unsigned  n_bits=8  bin_pt=2  align_bp=off  latency=1  explicit_period=off  period=1  en=off  dbl_ovrd=off  show_param=off
      settings: xl_area=[0, 0, 0, 0, 0, 0, 0]
  Logical{3,6,9,12} (4 alike) : xbsIndex_r3/Logical  logical_function=AND  inputs=4  precision=Full  arith_type=Unsigned  n_bits=8  bin_pt=2  align_bp=off  latency=1  explicit_period=off  period=1  en=off  dbl_ovrd=off  show_param=off
      settings: xl_area=[0, 0, 0, 0, 0, 0, 0]
  Logical13 : xbsIndex_r3/Logical  logical_function=AND  inputs=2  precision=Full  arith_type=Unsigned  n_bits=8  bin_pt=2  align_bp=off  latency=1  explicit_period=off  period=1  en=off  dbl_ovrd=off  show_param=off
      settings: xl_area=[0, 0, 0, 0, 0, 0, 0]
  Mux{,1..3} (4 alike) : xbsIndex_r3/Mux  inputs=2  precision=Full  arith_type="Signed  (2's comp)"  n_bits=8  bin_pt=2  quantization=Truncate  overflow=Wrap  latency=1  explicit_period=off  period=1  en=off  dbl_ovrd=off  show_param=off  mux_type=off  use_rpm=off  gen_core=off
      settings: xl_area=[0, 0, 0, 0, 0, 0, 0]
  Scale{,1..3} (4 alike) : xbsIndex_r3/Scale  scale_factor=-1  explicit_period=off  period=1  dbl_ovrd=off
  Slice{1,5,9,13} (4 alike) : xbsIndex_r3/Slice  mode=Upper Bit Location + Width  nbits=1  bit1=0  base1=MSB of Input  bit0=0  base0=LSB of Input  boolean_output=on  explicit_period=off  period=1  dbl_ovrd=off
  Slice{2,6,10,14} (4 alike) : xbsIndex_r3/Slice  mode=Upper Bit Location + Width  nbits=1  bit1=-1  base1=MSB of Input  bit0=0  base0=LSB of Input  boolean_output=on  explicit_period=off  period=1  dbl_ovrd=off
  Slice{3,7,11,15} (4 alike) : xbsIndex_r3/Slice  mode=Upper Bit Location + Width  nbits=1  bit1=-2  base1=MSB of Input  bit0=0  base0=LSB of Input  boolean_output=on  explicit_period=off  period=1  dbl_ovrd=off
  Slice{4,8,12,16} (4 alike) : xbsIndex_r3/Slice  mode=Upper Bit Location + Width  nbits=1  bit1=-3  base1=MSB of Input  bit0=0  base0=LSB of Input  boolean_output=on  explicit_period=off  period=1  dbl_ovrd=off
  ri_to_c : casper_library/Misc/ri_to_c
  ri_to_c1 : casper_library/Misc/ri_to_c
  twiddle : Subsystem  BlockChoice=twiddle_general_3mult
      link override twiddle_general_3mult: Coeffs=[exp(-2*pi*1j*(bit_rev(Coeffs, FFTSize-1))/2^FFTSize)]  StepPeriod=0  BitWidth=18  add_latency=3  mult_latency=4  bram_latency=3
      link override twiddle_general_3mult/coeff_gen: BlockChoice=br_coeff_gen
      link override twiddle_general_3mult/coeff_gen/br_coeff_gen: Coeffs=[1 2 3 4 5 6 7]  StepPeriod=4  BitWidth=10  bram_latency=6
      link override twiddle_general_3mult/coeff_gen/br_coeff_gen/ROM: distributed_mem=off
      link override twiddle_general_3mult/coeff_gen/br_coeff_gen/ROM1: distributed_mem=off
      link override twiddle_general_3mult/coeff_gen/static_coeff_gen/Constant: equ=P=C
      link override twiddle_general_3mult/coeff_gen/static_coeff_gen/Constant1: equ=P=C
      settings: AttributesFormatString=%<BlockChoice>  TemplateBlock=casper_library/FFTs/Twiddle/twiddle  MemberBlocks=twiddle_coeff_0,twiddle_coeff_1,twiddle_general_3mult,twiddle_general_4mult,twiddle_stage_2
  a+bw : Outport
  a-bw : Outport  Port=2
  of : Outport  Port=3
  sync_out : Outport  Port=4
  wires:
  Inverter/1 -> Logical13/1
  Logical13/1 -> of/1
  Logical/1 -> Logical13/2
  Delay3/1 -> Inverter/1, Mux3/1, Mux2/1, Mux1/1, Mux/1
  Logical7/1 -> Logical/3
  AddSub3/1 -> Scale3/1, Mux3/2
  Logical10/1 -> Logical/4
  Logical11/1 -> Logical10/2
  Logical12/1 -> Logical10/1
  Slice16/1 -> Logical11/3, Logical11/4, Logical12/4
  Slice15/1 -> Logical12/3
  Slice14/1 -> Logical11/2, Logical12/2
  Slice13/1 -> Logical11/1, Logical12/1
  Convert3/1 -> ri_to_c1/2
  Scale3/1 -> Mux3/3
  Mux3/1 -> Slice16/1, Slice15/1, Slice14/1, Slice13/1, Convert3/1
  AddSub2/1 -> Scale2/1, Mux2/2
  Logical8/1 -> Logical7/2
  Logical9/1 -> Logical7/1
  Slice12/1 -> Logical8/4, Logical9/4
  Slice11/1 -> Logical8/3, Logical9/3
  Slice10/1 -> Logical8/2, Logical9/2
  Slice9/1 -> Logical8/1, Logical9/1
  Convert2/1 -> ri_to_c1/1
  Scale2/1 -> Mux2/3
  Mux2/1 -> Slice12/1, Slice11/1, Slice10/1, Slice9/1, Convert2/1
  Logical4/1 -> Logical/2
  Logical5/1 -> Logical4/2
  Logical6/1 -> Logical4/1
  Slice8/1 -> Logical5/3, Logical5/4, Logical6/4
  Slice7/1 -> Logical6/3
  Slice6/1 -> Logical5/2, Logical6/2
  Slice5/1 -> Logical5/1, Logical6/1
  Convert1/1 -> ri_to_c/2
  Scale1/1 -> Mux1/3
  Mux1/1 -> Slice8/1, Slice7/1, Slice6/1, Slice5/1, Convert1/1
  Logical1/1 -> Logical/1
  Logical2/1 -> Logical1/2
  Logical3/1 -> Logical1/1
  Slice4/1 -> Logical2/4, Logical3/4
  Slice3/1 -> Logical2/3, Logical3/3
  Slice2/1 -> Logical2/2, Logical3/2
  Slice1/1 -> Logical2/1, Logical3/1
  Convert/1 -> ri_to_c/1
  Scale/1 -> Mux/3
  Mux/1 -> Slice4/1, Slice3/1, Slice2/1, Slice1/1, Convert/1
  shift/1 -> Delay3/1
  AddSub1/1 -> Scale1/1, Mux1/2
  AddSub/1 -> Scale/1, Mux/2
  Delay/1 -> sync_out/1
  ri_to_c1/1 -> a-bw/1
  ri_to_c/1 -> a+bw/1
  a/1 -> twiddle/1(a)
  b/1 -> twiddle/2(b)
  sync/1 -> twiddle/3(sync)
  twiddle/1(a_re) -> AddSub/1, AddSub2/1
  twiddle/2(a_im) -> AddSub1/1, AddSub3/1
  twiddle/3(bw_re) -> AddSub/2, AddSub2/2
  twiddle/4(bw_im) -> AddSub1/2, AddSub3/2
  twiddle/5(sync_out) -> Delay/1

== system dig_int_kurt/fft/fft_biplex0/biplex_core/fft_stage_10/delay_b ==
  In1 : Inport  Port=1  LatchInput=off
  delay_slr : casper_library/Delays/delay_slr  DelayLen=2^(FFTSize-FFTStage)
  Out1 : Outport
  wires:
  In1/1 -> delay_slr/1
  delay_slr/1 -> Out1/1

== system dig_int_kurt/fft/fft_biplex0/biplex_core/fft_stage_10/delay_f ==
  In1 : Inport  Port=1  LatchInput=off
  delay_slr : casper_library/Delays/delay_slr  DelayLen=2^(FFTSize-FFTStage)
  Out1 : Outport
  wires:
  In1/1 -> delay_slr/1
  delay_slr/1 -> Out1/1

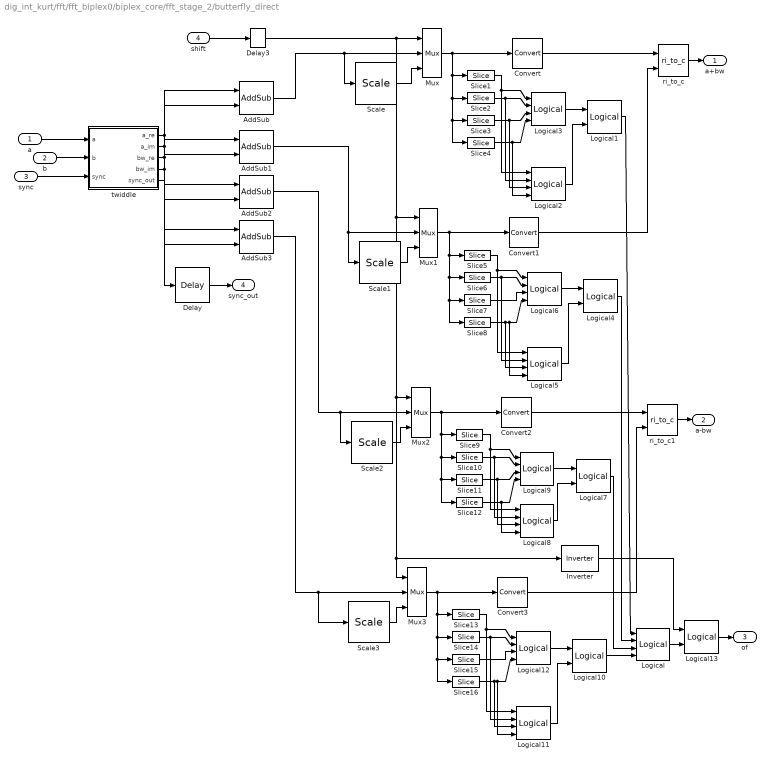
== system dig_int_kurt/fft/fft_biplex0/biplex_core/fft_stage_2/butterfly_direct ==
  a : Inport  Port=1  LatchInput=off
  b : Inport  Port=2  LatchInput=off
  sync : Inport  Port=3  LatchInput=off
  shift : Inport  Port=4  LatchInput=off
  AddSub : xbsIndex_r3/AddSub  mode=Addition  precision=Full  arith_type=Unsigned  n_bits=8  bin_pt=2  quantization=Truncate  overflow=Wrap  latency=add_latency  explicit_period=off  period=1  use_carryin=off  use_carryout=off  en=off  dbl_ovrd=off  show_param=on  use_core=on  pipeline=on  use_rpm=on  gen_core=on
      settings: xl_area=[0, 0, 0, 0, 0, 0, 0]
  AddSub1 : xbsIndex_r3/AddSub  mode=Addition  precision=Full  arith_type=Unsigned  n_bits=8  bin_pt=2  quantization=Truncate  overflow=Wrap  latency=add_latency  explicit_period=off  period=1  use_carryin=off  use_carryout=off  en=off  dbl_ovrd=off  show_param=on  use_core=on  pipeline=on  use_rpm=on  gen_core=on
      settings: xl_area=[0, 0, 0, 0, 0, 0, 0]
  AddSub2 : xbsIndex_r3/AddSub  mode=Subtraction  precision=Full  arith_type=Unsigned  n_bits=8  bin_pt=2  quantization=Truncate  overflow=Wrap  latency=add_latency  explicit_period=off  period=1  use_carryin=off  use_carryout=off  en=off  dbl_ovrd=off  show_param=on  use_core=on  pipeline=on  use_rpm=on  gen_core=on
      settings: xl_area=[0, 0, 0, 0, 0, 0, 0]
  AddSub3 : xbsIndex_r3/AddSub  mode=Subtraction  precision=Full  arith_type=Unsigned  n_bits=8  bin_pt=2  quantization=Truncate  overflow=Wrap  latency=add_latency  explicit_period=off  period=1  use_carryin=off  use_carryout=off  en=off  dbl_ovrd=off  show_param=on  use_core=on  pipeline=on  use_rpm=on  gen_core=on
      settings: xl_area=[0, 0, 0, 0, 0, 0, 0]
  Convert{,1..3} (4 alike) : xbsIndex_r3/Convert  arith_type="Signed  (2's comp)"  n_bits=BitWidth  bin_pt=BitWidth-1  quantization=Truncate  overflow=Wrap  latency=add_latency  explicit_period=off  period=1  dbl_ovrd=off  show_param=off  inserted_by_tool=off  pipeline=off
      settings: xl_area=[0, 0, 0, 0, 0, 0, 0]
  Delay : xbsIndex_r3/Delay  latency=2 * add_latency + 1  reg_retiming=off  explicit_period=off  period=1  en=off  accept_only_valid=off  init_zero=on  dbl_ovrd=off  show_param=off
      settings: xl_area=[0, 0, 0, 0, 0, 0, 0]
  Delay3 : xbsIndex_r3/Delay  latency=1  reg_retiming=off  explicit_period=off  period=1  en=off  accept_only_valid=off  init_zero=on  dbl_ovrd=off  show_param=off
      settings: xl_area=[0, 0, 0, 0, 0, 0, 0]
  Inverter : xbsIndex_r3/Inverter  latency=0  explicit_period=off  period=1  en=off  dbl_ovrd=off  show_param=off
      settings: xl_area=[0, 0, 0, 0, 0, 0, 0]
  Logical : xbsIndex_r3/Logical  logical_function=OR  inputs=4  precision=Full  arith_type=Unsigned  n_bits=8  bin_pt=2  align_bp=on  latency=1  explicit_period=off  period=1  en=off  dbl_ovrd=off  show_param=off
      settings: xl_area=[0, 0, 0, 0, 0, 0, 0]
  Logical{1,4,7,10} (4 alike) : xbsIndex_r3/Logical  logical_function=OR  inputs=2  precision=Full  arith_type=Unsigned  n_bits=8  bin_pt=2  align_bp=off  latency=1  explicit_period=off  period=1  en=off  dbl_ovrd=off  show_param=off
      settings: xl_area=[0, 0, 0, 0, 0, 0, 0]
  Logical{2,5,8,11} (4 alike) : xbsIndex_r3/Logical  logical_function=NOR  inputs=4  precision=Full  arith_type=Unsigned  n_bits=8  bin_pt=2  align_bp=off  latency=1  explicit_period=off  period=1  en=off  dbl_ovrd=off  show_param=off
      settings: xl_area=[0, 0, 0, 0, 0, 0, 0]
  Logical{3,6,9,12} (4 alike) : xbsIndex_r3/Logical  logical_function=AND  inputs=4  precision=Full  arith_type=Unsigned  n_bits=8  bin_pt=2  align_bp=off  latency=1  explicit_period=off  period=1  en=off  dbl_ovrd=off  show_param=off
      settings: xl_area=[0, 0, 0, 0, 0, 0, 0]
  Logical13 : xbsIndex_r3/Logical  logical_function=AND  inputs=2  precision=Full  arith_type=Unsigned  n_bits=8  bin_pt=2  align_bp=off  latency=1  explicit_period=off  period=1  en=off  dbl_ovrd=off  show_param=off
      settings: xl_area=[0, 0, 0, 0, 0, 0, 0]
  Mux{,1..3} (4 alike) : xbsIndex_r3/Mux  inputs=2  precision=Full  arith_type="Signed  (2's comp)"  n_bits=8  bin_pt=2  quantization=Truncate  overflow=Wrap  latency=1  explicit_period=off  period=1  en=off  dbl_ovrd=off  show_param=off  mux_type=off  use_rpm=off  gen_core=off
      settings: xl_area=[0, 0, 0, 0, 0, 0, 0]
  Scale{,1..3} (4 alike) : xbsIndex_r3/Scale  scale_factor=-1  explicit_period=off  period=1  dbl_ovrd=off
  Slice{1,5,9,13} (4 alike) : xbsIndex_r3/Slice  mode=Upper Bit Location + Width  nbits=1  bit1=0  base1=MSB of Input  bit0=0  base0=LSB of Input  boolean_output=on  explicit_period=off  period=1  dbl_ovrd=off
  Slice{2,6,10,14} (4 alike) : xbsIndex_r3/Slice  mode=Upper Bit Location + Width  nbits=1  bit1=-1  base1=MSB of Input  bit0=0  base0=LSB of Input  boolean_output=on  explicit_period=off  period=1  dbl_ovrd=off
  Slice{3,7,11,15} (4 alike) : xbsIndex_r3/Slice  mode=Upper Bit Location + Width  nbits=1  bit1=-2  base1=MSB of Input  bit0=0  base0=LSB of Input  boolean_output=on  explicit_period=off  period=1  dbl_ovrd=off
  Slice{4,8,12,16} (4 alike) : xbsIndex_r3/Slice  mode=Upper Bit Location + Width  nbits=1  bit1=-3  base1=MSB of Input  bit0=0  base0=LSB of Input  boolean_output=on  explicit_period=off  period=1  dbl_ovrd=off
  ri_to_c : casper_library/Misc/ri_to_c
  ri_to_c1 : casper_library/Misc/ri_to_c
  twiddle : Subsystem  BlockChoice=twiddle_stage_2
      link override twiddle_general_3mult: Coeffs="[1+0i           6.1232e-017-1i          ]"  StepPeriod=9  BitWidth=18  add_latency=2  mult_latency=3  bram_latency=2
      link override twiddle_general_3mult/coeff_gen: BlockChoice=br_coeff_gen
      link override twiddle_general_3mult/coeff_gen/br_coeff_gen: Coeffs=[1 2 3 4 5 6 7]  StepPeriod=4  BitWidth=10  bram_latency=6
      link override twiddle_general_3mult/coeff_gen/br_coeff_gen/ROM: distributed_mem=off
      link override twiddle_general_3mult/coeff_gen/br_coeff_gen/ROM1: distributed_mem=off
      link override twiddle_stage_2: FFTSize=10  BitWidth=18  add_latency=3  mult_latency=4  bram_latency=3
      settings: AttributesFormatString=%<BlockChoice>  TemplateBlock=casper_library/FFTs/Twiddle/twiddle  MemberBlocks=twiddle_coeff_0,twiddle_coeff_1,twiddle_general_3mult,twiddle_general_4mult,twiddle_stage_2
  a+bw : Outport
  a-bw : Outport  Port=2
  of : Outport  Port=3
  sync_out : Outport  Port=4
  wires:
  Inverter/1 -> Logical13/1
  Logical13/1 -> of/1
  Logical/1 -> Logical13/2
  Delay3/1 -> Inverter/1, Mux3/1, Mux2/1, Mux1/1, Mux/1
  Logical7/1 -> Logical/3
  AddSub3/1 -> Scale3/1, Mux3/2
  Logical10/1 -> Logical/4
  Logical11/1 -> Logical10/2
  Logical12/1 -> Logical10/1
  Slice16/1 -> Logical11/3, Logical11/4, Logical12/4
  Slice15/1 -> Logical12/3
  Slice14/1 -> Logical11/2, Logical12/2
  Slice13/1 -> Logical11/1, Logical12/1
  Convert3/1 -> ri_to_c1/2
  Scale3/1 -> Mux3/3
  Mux3/1 -> Slice16/1, Slice15/1, Slice14/1, Slice13/1, Convert3/1
  AddSub2/1 -> Scale2/1, Mux2/2
  Logical8/1 -> Logical7/2
  Logical9/1 -> Logical7/1
  Slice12/1 -> Logical8/4, Logical9/4
  Slice11/1 -> Logical8/3, Logical9/3
  Slice10/1 -> Logical8/2, Logical9/2
  Slice9/1 -> Logical8/1, Logical9/1
  Convert2/1 -> ri_to_c1/1
  Scale2/1 -> Mux2/3
  Mux2/1 -> Slice12/1, Slice11/1, Slice10/1, Slice9/1, Convert2/1
  Logical4/1 -> Logical/2
  Logical5/1 -> Logical4/2
  Logical6/1 -> Logical4/1
  Slice8/1 -> Logical5/3, Logical5/4, Logical6/4
  Slice7/1 -> Logical6/3
  Slice6/1 -> Logical5/2, Logical6/2
  Slice5/1 -> Logical5/1, Logical6/1
  Convert1/1 -> ri_to_c/2
  Scale1/1 -> Mux1/3
  Mux1/1 -> Slice8/1, Slice7/1, Slice6/1, Slice5/1, Convert1/1
  Logical1/1 -> Logical/1
  Logical2/1 -> Logical1/2
  Logical3/1 -> Logical1/1
  Slice4/1 -> Logical2/4, Logical3/4
  Slice3/1 -> Logical2/3, Logical3/3
  Slice2/1 -> Logical2/2, Logical3/2
  Slice1/1 -> Logical2/1, Logical3/1
  Convert/1 -> ri_to_c/1
  Scale/1 -> Mux/3
  Mux/1 -> Slice4/1, Slice3/1, Slice2/1, Slice1/1, Convert/1
  shift/1 -> Delay3/1
  AddSub1/1 -> Scale1/1, Mux1/2
  AddSub/1 -> Scale/1, Mux/2
  Delay/1 -> sync_out/1
  ri_to_c1/1 -> a-bw/1
  ri_to_c/1 -> a+bw/1
  a/1 -> twiddle/1(a)
  b/1 -> twiddle/2(b)
  sync/1 -> twiddle/3(sync)
  twiddle/1(a_re) -> AddSub/1, AddSub2/1
  twiddle/2(a_im) -> AddSub1/1, AddSub3/1
  twiddle/3(bw_re) -> AddSub/2, AddSub2/2
  twiddle/4(bw_im) -> AddSub1/2, AddSub3/2
  twiddle/5(sync_out) -> Delay/1

== system dig_int_kurt/fft/fft_biplex0/biplex_core/fft_stage_2/delay_b ==
  In1 : Inport  Port=1  LatchInput=off
  delay_bram : casper_library/Delays/delay_bram  DelayLen=2^(FFTSize-FFTStage)  bram_latency=bram_latency
  Out1 : Outport
  wires:
  In1/1 -> delay_bram/1
  delay_bram/1 -> Out1/1
